simulink model "untitled"  (R2022b)
settings: Solver=VariableStepAuto  StartTime=0.0  StopTime=10.0  RelTol=1e-3
settings Model: Creator=admin  LastModifiedBy=admin

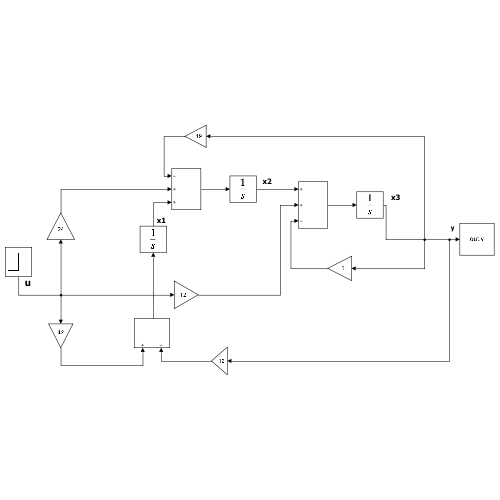
[thumbnail: Simulink's stored preview of the top-level diagram]
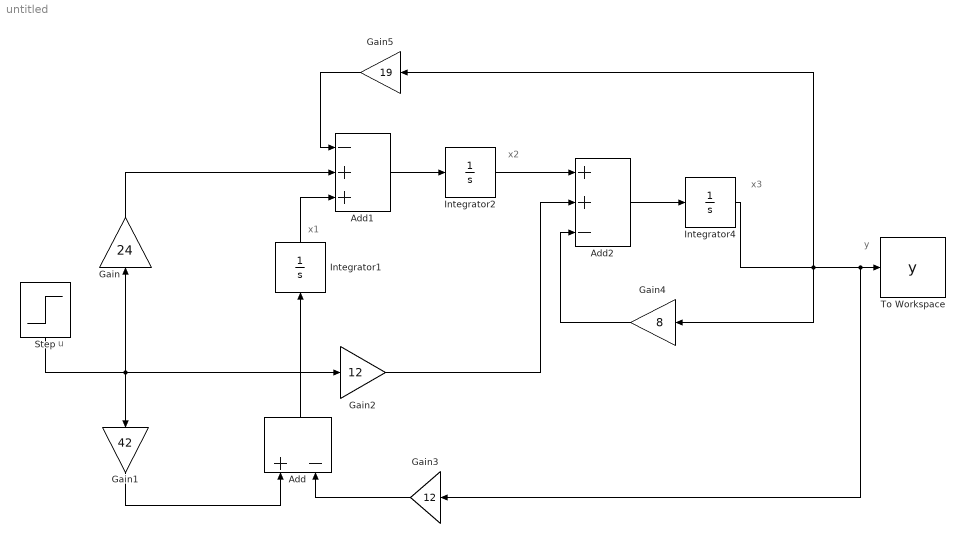
== system untitled ==
  note: y
  note: x3
  note: x2
  note: x1
  note: u
  Add : Sum  Inputs=+-
  Add1 : Sum  Inputs=-++
  Add2 : Sum  Inputs=++-
  Gain : Gain  Gain=24
  Gain1 : Gain  Gain=42
  Gain2 : Gain  Gain=12
  Gain3 : Gain  Gain=12
  Gain4 : Gain  Gain=8
  Gain5 : Gain  Gain=19
  Integrator1 : Integrator
  Integrator2 : Integrator
  Integrator4 : Integrator
  Step : Step  SampleTime=0
  To Workspace : ToWorkspace  VariableName=y  SaveFormat=Structure With Time  SampleTime=-1
  wires:
  Step/1 -> Gain1/1, Gain2/1, Gain/1
  Integrator1/1 -> Add1/3
  Gain/1 -> Add1/2
  Add1/1 -> Integrator2/1
  Integrator2/1 -> Add2/1
  Add/1 -> Integrator1/1
  Gain1/1 -> Add/1
  Gain5/1 -> Add1/1
  Gain4/1 -> Add2/3
  Gain2/1 -> Add2/2
  Add2/1 -> Integrator4/1
  Integrator4/1 -> Gain5/1, To Workspace/1, Gain3/1, Gain4/1
  Gain3/1 -> Add/2
